simulink model "lab1_analogs"  (R2020a)
settings: Solver=VariableStepAuto  StartTime=0.0  StopTime=100  RelTol=1e-3
settings Model: Creator=luis  LastModifiedBy=luis

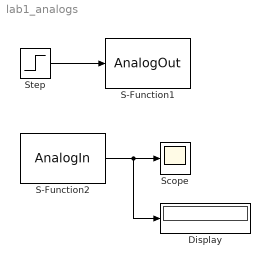
== system lab1_analogs ==
  Display : Display
  S-Function1 : S-Function  FunctionName=AnalogOut  SFunctionDeploymentMode=off  EnableBusSupport=off
  S-Function2 : S-Function  FunctionName=AnalogIn  SFunctionDeploymentMode=off  EnableBusSupport=off
  Scope : Scope
  Step : Step  After=5  SampleTime=0
  wires:
  Step/1 -> S-Function1/1
  S-Function2/1 -> Display/1, Scope/1
